simulink model "literal2_Simulink"  (R2026a)
settings: Solver=VariableStepAuto  StopTime=60
settings Model: Creator=Usuario  LastModifiedBy=Usuario

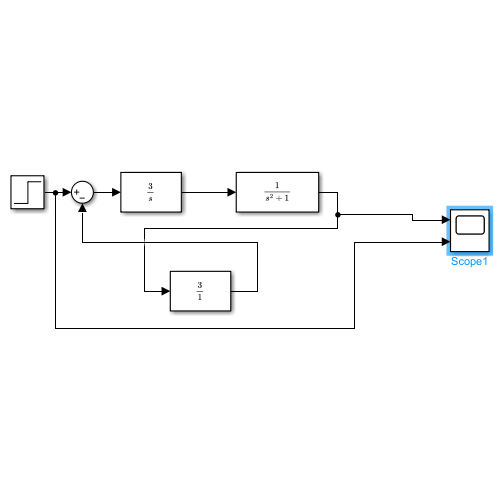
[thumbnail: Simulink's stored preview of the top-level diagram]
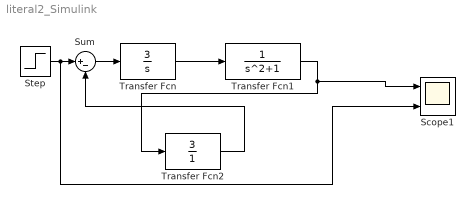
== system literal2_Simulink ==
  Scope1 : Scope  NumInputPorts=2
      settings: ActiveDisplayYMinimum=-6.2100219987487471  ActiveDisplayYMaximum=6.126656895539762
  Step : Step  SampleTime=0  ZeroCross=off
  Sum : Sum  Inputs=|+-
  Transfer Fcn : TransferFcn  Numerator=[3]  Denominator=[1 0]
  Transfer Fcn1 : TransferFcn  Denominator=[1 0 1]
  Transfer Fcn2 : TransferFcn  Numerator=[3]  Denominator=[1]
  wires:
  Step/1 -> Scope1/2, Sum/1
  Sum/1 -> Transfer Fcn/1
  Transfer Fcn/1 -> Transfer Fcn1/1
  Transfer Fcn2/1 -> Sum/2
  Transfer Fcn1/1 -> Scope1/1, Transfer Fcn2/1
